simulink model "AdderSubtractor"  (R2014a)
settings: Solver=ode45  StartTime=0.0  StopTime=10.0  RelTol=1e-3  EnableMultiTasking=on
libraries: hdlsllib x17
settings Model: Creator=downing.s  LastModifiedBy=you.r
settings OptimizationCC: SimCompilerOptimization=off
settings DebuggingCC: MergeDetectMultiDrivingBlocksExec=error  FcnCallInpInsideContextMsg=error  FrameProcessingCompatibilityMsg=error  SFExecutionAtInitializationDiag=none
settings HardwareCC: ProdBitPerSizeT=32  ProdBitPerPtrDiffT=32
settings RTWCC: RTWCompilerOptimization=off
settings ConfigComp: CovMetricSettings=dw  CovHtmlReporting=on  CovSaveCumulativeToWorkspaceVar=on  CovSaveSingleToWorkspaceVar=on  CovExternalEMLEnable=off  CovSFcnEnable=off

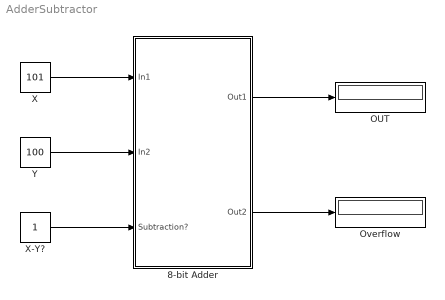
== system AdderSubtractor ==
  8-bit Adder : Subsystem
  OUT : Display
  Overflow : Display
  X : Constant  Value=101  OutDataTypeStr=int8  SampleTime=1
  X-Y? : Constant  OutDataTypeStr=boolean  SampleTime=1
  Y : Constant  Value=100  OutDataTypeStr=int8  SampleTime=1
  wires:
  X/1 -> 8-bit Adder/1(In1)
  Y/1 -> 8-bit Adder/2(In2)
  8-bit Adder/1(Out1) -> OUT/1
  8-bit Adder/2(Out2) -> Overflow/1
  X-Y?/1 -> 8-bit Adder/3("Subtraction? ")

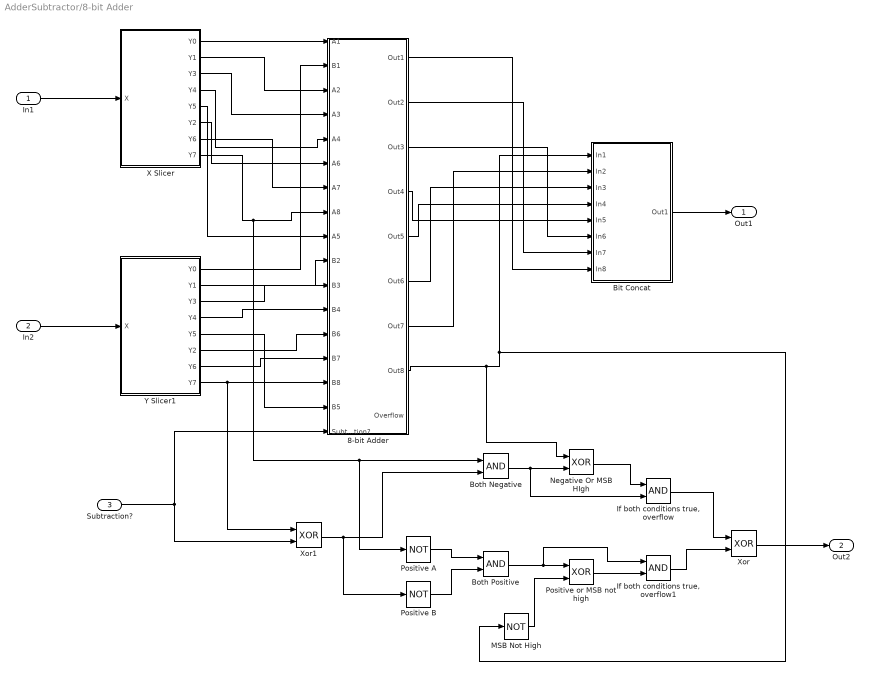
== system AdderSubtractor/8-bit Adder ==
  In1 : Inport
  In2 : Inport  Port=2
  "Subtraction? " : Inport  Port=3
  8-bit Adder : Subsystem
  Bit Concat : Subsystem
  Both Negative : Logic  AllPortsSameDT=off  OutDataTypeStr=boolean
  Both Positive : Logic  AllPortsSameDT=off  OutDataTypeStr=boolean
  "If both conditions true, overflow" : Logic  AllPortsSameDT=off  OutDataTypeStr=boolean
  "If both conditions true, overflow1" : Logic  AllPortsSameDT=off  OutDataTypeStr=boolean
  MSB Not High : Logic  Operator=NOT  AllPortsSameDT=off  OutDataTypeStr=boolean
  Negative Or MSB HIgh : Logic  Operator=XOR  AllPortsSameDT=off  OutDataTypeStr=boolean
  Positive A : Logic  Operator=NOT  AllPortsSameDT=off  OutDataTypeStr=boolean
  Positive B : Logic  Operator=NOT  AllPortsSameDT=off  OutDataTypeStr=boolean
  Positive or MSB not high : Logic  Operator=XOR  AllPortsSameDT=off  OutDataTypeStr=boolean
  X Slicer : Subsystem
  Xor : Logic  Operator=XOR  AllPortsSameDT=off  OutDataTypeStr=boolean
  Xor1 : Logic  Operator=XOR  AllPortsSameDT=off  OutDataTypeStr=boolean
  Y Slicer1 : Subsystem
  Out1 : Outport
  Out2 : Outport  Port=2
  wires:
  Bit Concat/1(Out1) -> Out1/1
  In1/1 -> X Slicer/1(X)
  In2/1 -> Y Slicer1/1(X)
  8-bit Adder/8(Out8) -> Negative Or MSB HIgh/1, MSB Not High/1, Bit Concat/1(In1)
  8-bit Adder/7(Out7) -> Bit Concat/2(In2)
  8-bit Adder/6(Out6) -> Bit Concat/3(In3)
  8-bit Adder/5(Out5) -> Bit Concat/4(In4)
  8-bit Adder/4(Out4) -> Bit Concat/5(In5)
  8-bit Adder/3(Out3) -> Bit Concat/6(In6)
  8-bit Adder/2(Out2) -> Bit Concat/7(In7)
  8-bit Adder/1(Out1) -> Bit Concat/8(In8)
  X Slicer/1(Y0) -> 8-bit Adder/1(A1)
  X Slicer/2(Y1) -> 8-bit Adder/3(A2)
  X Slicer/3(Y3) -> 8-bit Adder/4(A3)
  X Slicer/4(Y4) -> 8-bit Adder/5(A4)
  X Slicer/5(Y5) -> 8-bit Adder/9(A5)
  X Slicer/6(Y2) -> 8-bit Adder/6(A6)
  X Slicer/7(Y6) -> 8-bit Adder/7(A7)
  Y Slicer1/1(Y0) -> 8-bit Adder/2(B1)
  Y Slicer1/2(Y1) -> 8-bit Adder/10(B2)
  Y Slicer1/3(Y3) -> 8-bit Adder/11(B3)
  Y Slicer1/4(Y4) -> 8-bit Adder/12(B4)
  Y Slicer1/5(Y5) -> 8-bit Adder/16(B5)
  Y Slicer1/6(Y2) -> 8-bit Adder/13(B6)
  Y Slicer1/7(Y6) -> 8-bit Adder/14(B7)
  Y Slicer1/8(Y7) -> Xor1/1, 8-bit Adder/15(B8)
  Both Negative/1 -> "If both conditions true, overflow"/2, Negative Or MSB HIgh/2
  Negative Or MSB HIgh/1 -> "If both conditions true, overflow"/1
  X Slicer/8(Y7) -> Positive A/1, Both Negative/1, 8-bit Adder/8(A8)
  Positive A/1 -> Both Positive/1
  Positive B/1 -> Both Positive/2
  Both Positive/1 -> "If both conditions true, overflow1"/1, Positive or MSB not high/1
  MSB Not High/1 -> Positive or MSB not high/2
  Positive or MSB not high/1 -> "If both conditions true, overflow1"/2
  Xor/1 -> Out2/1
  "If both conditions true, overflow1"/1 -> Xor/2
  "If both conditions true, overflow"/1 -> Xor/1
  "Subtraction? "/1 -> 8-bit Adder/17(Subtraction?), Xor1/2
  Xor1/1 -> Positive B/1, Both Negative/2

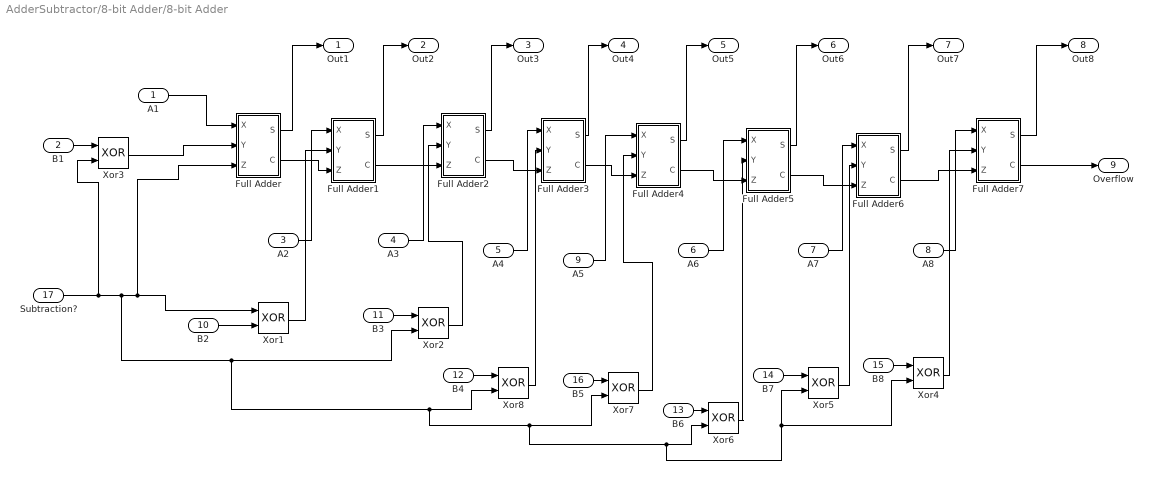
== system AdderSubtractor/8-bit Adder/8-bit Adder ==
  A1 : Inport
  B1 : Inport  Port=2
  A2 : Inport  Port=3
  A3 : Inport  Port=4
  A4 : Inport  Port=5
  A6 : Inport  Port=6
  A7 : Inport  Port=7
  A8 : Inport  Port=8
  A5 : Inport  Port=9
  B2 : Inport  Port=10
  B3 : Inport  Port=11
  B4 : Inport  Port=12
  B6 : Inport  Port=13
  B7 : Inport  Port=14
  B8 : Inport  Port=15
  B5 : Inport  Port=16
  Subtraction? : Inport  Port=17  OutDataTypeStr=boolean
  Full Adder : Subsystem
  Full Adder1 : Subsystem
  Full Adder2 : Subsystem
  Full Adder3 : Subsystem
  Full Adder4 : Subsystem
  Full Adder5 : Subsystem
  Full Adder6 : Subsystem
  Full Adder7 : Subsystem
  Xor{1..8} (8 alike) : Logic  Operator=XOR  AllPortsSameDT=off  OutDataTypeStr=boolean
  Out1 : Outport  OutDataTypeStr=boolean
  Out2 : Outport  Port=2  OutDataTypeStr=boolean
  Out3 : Outport  Port=3  OutDataTypeStr=boolean
  Out4 : Outport  Port=4  OutDataTypeStr=boolean
  Out5 : Outport  Port=5  OutDataTypeStr=boolean
  Out6 : Outport  Port=6  OutDataTypeStr=boolean
  Out7 : Outport  Port=7  OutDataTypeStr=boolean
  Out8 : Outport  Port=8  OutDataTypeStr=boolean
  Overflow : Outport  Port=9  OutDataTypeStr=boolean
  wires:
  Full Adder7/2(C) -> Overflow/1
  Full Adder5/2(C) -> Full Adder6/3(Z)
  Full Adder7/1(S) -> Out8/1
  Full Adder4/2(C) -> Full Adder5/3(Z)
  Full Adder/2(C) -> Full Adder1/3(Z)
  Full Adder6/2(C) -> Full Adder7/3(Z)
  Full Adder6/1(S) -> Out7/1
  Full Adder2/2(C) -> Full Adder3/3(Z)
  Full Adder4/1(S) -> Out5/1
  A2/1 -> Full Adder1/1(X)
  A5/1 -> Full Adder4/1(X)
  Full Adder1/1(S) -> Out2/1
  A7/1 -> Full Adder6/1(X)
  Full Adder5/1(S) -> Out6/1
  A1/1 -> Full Adder/1(X)
  A8/1 -> Full Adder7/1(X)
  A6/1 -> Full Adder5/1(X)
  A4/1 -> Full Adder3/1(X)
  Full Adder3/1(S) -> Out4/1
  Full Adder/1(S) -> Out1/1
  Full Adder1/2(C) -> Full Adder2/3(Z)
  A3/1 -> Full Adder2/1(X)
  Full Adder3/2(C) -> Full Adder4/3(Z)
  Full Adder2/1(S) -> Out3/1
  B2/1 -> Xor1/2
  Subtraction?/1 -> Xor3/2, Xor4/2, Xor5/2, Xor6/2, Xor7/2, Xor8/2, Xor2/2, Full Adder/3(Z), Xor1/1
  Xor1/1 -> Full Adder1/2(Y)
  Xor2/1 -> Full Adder2/2(Y)
  B3/1 -> Xor2/1
  B4/1 -> Xor8/1
  Xor8/1 -> Full Adder3/2(Y)
  B5/1 -> Xor7/1
  Xor7/1 -> Full Adder4/2(Y)
  B6/1 -> Xor6/1
  Xor6/1 -> Full Adder5/2(Y)
  B7/1 -> Xor5/1
  Xor5/1 -> Full Adder6/2(Y)
  Xor4/1 -> Full Adder7/2(Y)
  B8/1 -> Xor4/1
  Xor3/1 -> Full Adder/2(Y)
  B1/1 -> Xor3/1

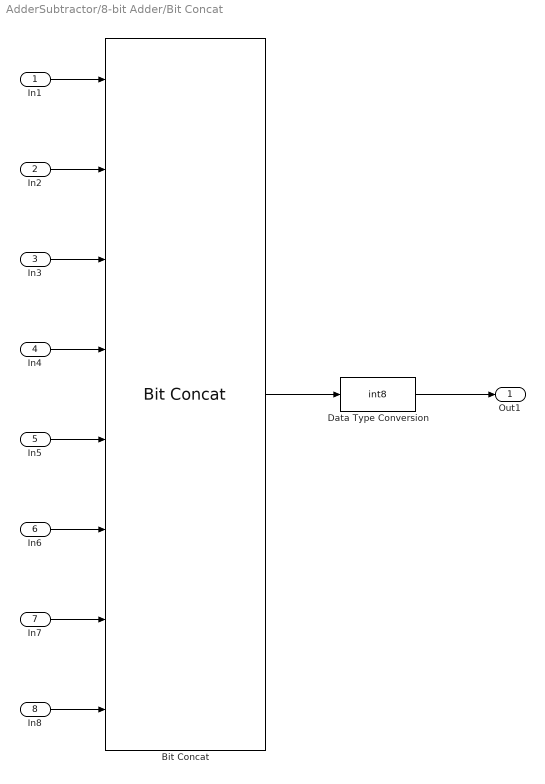
== system AdderSubtractor/8-bit Adder/Bit Concat ==
  In1 : Inport
  In2 : Inport  Port=2
  In3 : Inport  Port=3
  In4 : Inport  Port=4
  In5 : Inport  Port=5
  In6 : Inport  Port=6
  In7 : Inport  Port=7
  In8 : Inport  Port=8
  Bit Concat : hdlsllib/HDL Operations/Bit Concat  numInputs=8
  Data Type Conversion : DataTypeConversion  OutDataTypeStr=int8
  Out1 : Outport
  wires:
  Data Type Conversion/1 -> Out1/1
  In4/1 -> Bit Concat/4
  In1/1 -> Bit Concat/1
  In2/1 -> Bit Concat/2
  In5/1 -> Bit Concat/5
  In6/1 -> Bit Concat/6
  In7/1 -> Bit Concat/7
  In8/1 -> Bit Concat/8
  In3/1 -> Bit Concat/3
  Bit Concat/1 -> Data Type Conversion/1

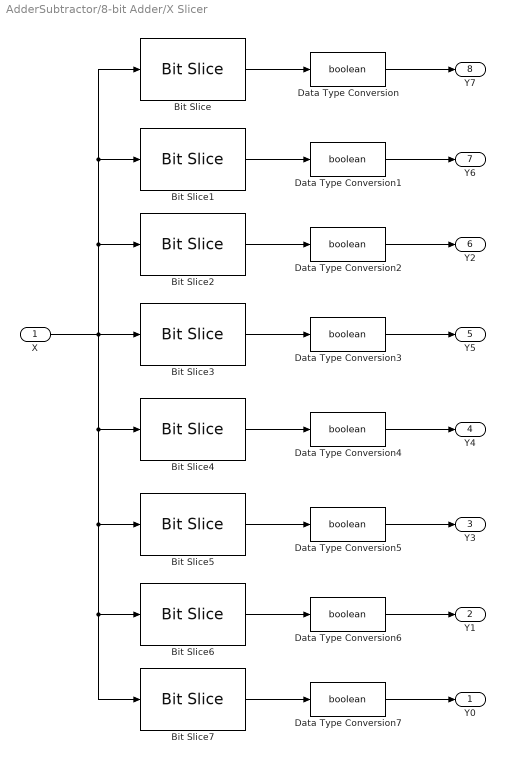
== system AdderSubtractor/8-bit Adder/X Slicer ==
  X : Inport  OutDataTypeStr=int8  SampleTime=1
  Bit Slice : hdlsllib/HDL Operations/Bit Slice  lidx=7  ridx=7
  Bit Slice1 : hdlsllib/HDL Operations/Bit Slice  lidx=6  ridx=6
  Bit Slice2 : hdlsllib/HDL Operations/Bit Slice  lidx=5  ridx=5
  Bit Slice3 : hdlsllib/HDL Operations/Bit Slice  lidx=4  ridx=4
  Bit Slice4 : hdlsllib/HDL Operations/Bit Slice  lidx=3  ridx=3
  Bit Slice5 : hdlsllib/HDL Operations/Bit Slice  lidx=2  ridx=2
  Bit Slice6 : hdlsllib/HDL Operations/Bit Slice  lidx=1  ridx=1
  Bit Slice7 : hdlsllib/HDL Operations/Bit Slice  lidx=0  ridx=0
  Data Type Conversion{,1..7} (8 alike) : DataTypeConversion  OutDataTypeStr=boolean
  Y0 : Outport
  Y1 : Outport  Port=2
  Y3 : Outport  Port=3
  Y4 : Outport  Port=4
  Y5 : Outport  Port=5
  Y2 : Outport  Port=6
  Y6 : Outport  Port=7
  Y7 : Outport  Port=8
  wires:
  X/1 -> Bit Slice4/1, Bit Slice5/1, Bit Slice6/1, Bit Slice7/1, Bit Slice3/1, Bit Slice2/1, Bit Slice1/1, Bit Slice/1
  Data Type Conversion/1 -> Y7/1
  Data Type Conversion1/1 -> Y6/1
  Bit Slice2/1 -> Data Type Conversion2/1
  Bit Slice3/1 -> Data Type Conversion3/1
  Bit Slice4/1 -> Data Type Conversion4/1
  Data Type Conversion6/1 -> Y1/1
  Bit Slice/1 -> Data Type Conversion/1
  Bit Slice1/1 -> Data Type Conversion1/1
  Bit Slice6/1 -> Data Type Conversion6/1
  Data Type Conversion7/1 -> Y0/1
  Bit Slice7/1 -> Data Type Conversion7/1
  Bit Slice5/1 -> Data Type Conversion5/1
  Data Type Conversion2/1 -> Y2/1
  Data Type Conversion3/1 -> Y5/1
  Data Type Conversion4/1 -> Y4/1
  Data Type Conversion5/1 -> Y3/1

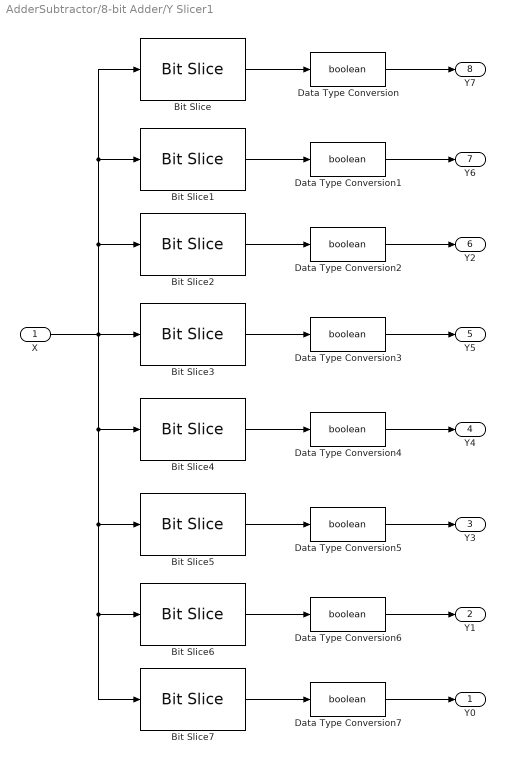
== system AdderSubtractor/8-bit Adder/Y Slicer1 ==
  X : Inport  OutDataTypeStr=int8  SampleTime=1
  Bit Slice : hdlsllib/HDL Operations/Bit Slice  lidx=7  ridx=7
  Bit Slice1 : hdlsllib/HDL Operations/Bit Slice  lidx=6  ridx=6
  Bit Slice2 : hdlsllib/HDL Operations/Bit Slice  lidx=5  ridx=5
  Bit Slice3 : hdlsllib/HDL Operations/Bit Slice  lidx=4  ridx=4
  Bit Slice4 : hdlsllib/HDL Operations/Bit Slice  lidx=3  ridx=3
  Bit Slice5 : hdlsllib/HDL Operations/Bit Slice  lidx=2  ridx=2
  Bit Slice6 : hdlsllib/HDL Operations/Bit Slice  lidx=1  ridx=1
  Bit Slice7 : hdlsllib/HDL Operations/Bit Slice  lidx=0  ridx=0
  Data Type Conversion{,1..7} (8 alike) : DataTypeConversion  OutDataTypeStr=boolean
  Y0 : Outport
  Y1 : Outport  Port=2
  Y3 : Outport  Port=3
  Y4 : Outport  Port=4
  Y5 : Outport  Port=5
  Y2 : Outport  Port=6
  Y6 : Outport  Port=7
  Y7 : Outport  Port=8
  wires:
  X/1 -> Bit Slice4/1, Bit Slice5/1, Bit Slice6/1, Bit Slice7/1, Bit Slice3/1, Bit Slice2/1, Bit Slice1/1, Bit Slice/1
  Data Type Conversion/1 -> Y7/1
  Data Type Conversion1/1 -> Y6/1
  Bit Slice2/1 -> Data Type Conversion2/1
  Bit Slice3/1 -> Data Type Conversion3/1
  Bit Slice4/1 -> Data Type Conversion4/1
  Data Type Conversion6/1 -> Y1/1
  Bit Slice/1 -> Data Type Conversion/1
  Bit Slice1/1 -> Data Type Conversion1/1
  Bit Slice6/1 -> Data Type Conversion6/1
  Data Type Conversion7/1 -> Y0/1
  Bit Slice7/1 -> Data Type Conversion7/1
  Bit Slice5/1 -> Data Type Conversion5/1
  Data Type Conversion2/1 -> Y2/1
  Data Type Conversion3/1 -> Y5/1
  Data Type Conversion4/1 -> Y4/1
  Data Type Conversion5/1 -> Y3/1

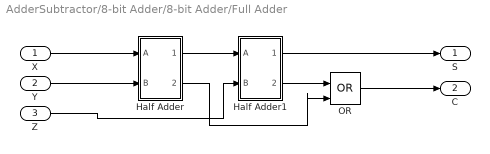
== system AdderSubtractor/8-bit Adder/8-bit Adder/Full Adder ==
  X : Inport
  Y : Inport  Port=2
  Z : Inport  Port=3
  Half Adder : Subsystem
  Half Adder1 : Subsystem
  OR : Logic  Operator=OR  IconShape=distinctive  AllPortsSameDT=off  OutDataTypeStr=boolean
  S : Outport
  C : Outport  Port=2
  wires:
  Half Adder1/1(Sum) -> S/1
  Half Adder/1(Sum) -> Half Adder1/1(A)
  Half Adder/2(Carry) -> OR/2
  X/1 -> Half Adder/1(A)
  Z/1 -> Half Adder1/2(B)
  OR/1 -> C/1
  Y/1 -> Half Adder/2(B)
  Half Adder1/2(Carry) -> OR/1

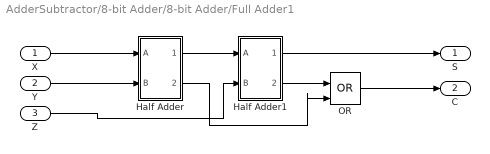
== system AdderSubtractor/8-bit Adder/8-bit Adder/Full Adder1 ==
  X : Inport
  Y : Inport  Port=2
  Z : Inport  Port=3
  Half Adder : Subsystem
  Half Adder1 : Subsystem
  OR : Logic  Operator=OR  IconShape=distinctive  AllPortsSameDT=off  OutDataTypeStr=boolean
  S : Outport
  C : Outport  Port=2
  wires:
  Half Adder1/1(Sum) -> S/1
  Half Adder/1(Sum) -> Half Adder1/1(A)
  Half Adder/2(Carry) -> OR/2
  X/1 -> Half Adder/1(A)
  Z/1 -> Half Adder1/2(B)
  OR/1 -> C/1
  Y/1 -> Half Adder/2(B)
  Half Adder1/2(Carry) -> OR/1

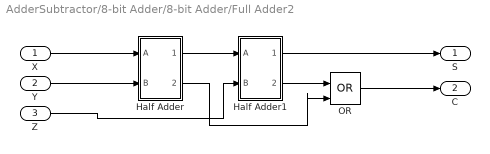
== system AdderSubtractor/8-bit Adder/8-bit Adder/Full Adder2 ==
  X : Inport
  Y : Inport  Port=2
  Z : Inport  Port=3
  Half Adder : Subsystem
  Half Adder1 : Subsystem
  OR : Logic  Operator=OR  IconShape=distinctive  AllPortsSameDT=off  OutDataTypeStr=boolean
  S : Outport
  C : Outport  Port=2
  wires:
  Half Adder1/1(Sum) -> S/1
  Half Adder/1(Sum) -> Half Adder1/1(A)
  Half Adder/2(Carry) -> OR/2
  X/1 -> Half Adder/1(A)
  Z/1 -> Half Adder1/2(B)
  OR/1 -> C/1
  Y/1 -> Half Adder/2(B)
  Half Adder1/2(Carry) -> OR/1

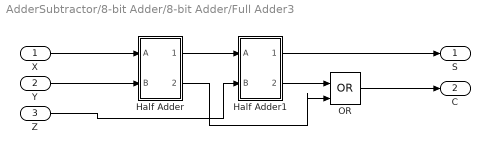
== system AdderSubtractor/8-bit Adder/8-bit Adder/Full Adder3 ==
  X : Inport
  Y : Inport  Port=2
  Z : Inport  Port=3
  Half Adder : Subsystem
  Half Adder1 : Subsystem
  OR : Logic  Operator=OR  IconShape=distinctive  AllPortsSameDT=off  OutDataTypeStr=boolean
  S : Outport
  C : Outport  Port=2
  wires:
  Half Adder1/1(Sum) -> S/1
  Half Adder/1(Sum) -> Half Adder1/1(A)
  Half Adder/2(Carry) -> OR/2
  X/1 -> Half Adder/1(A)
  Z/1 -> Half Adder1/2(B)
  OR/1 -> C/1
  Y/1 -> Half Adder/2(B)
  Half Adder1/2(Carry) -> OR/1

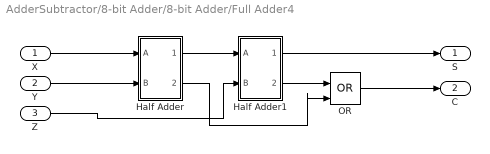
== system AdderSubtractor/8-bit Adder/8-bit Adder/Full Adder4 ==
  X : Inport
  Y : Inport  Port=2
  Z : Inport  Port=3
  Half Adder : Subsystem
  Half Adder1 : Subsystem
  OR : Logic  Operator=OR  IconShape=distinctive  AllPortsSameDT=off  OutDataTypeStr=boolean
  S : Outport
  C : Outport  Port=2
  wires:
  Half Adder1/1(Sum) -> S/1
  Half Adder/1(Sum) -> Half Adder1/1(A)
  Half Adder/2(Carry) -> OR/2
  X/1 -> Half Adder/1(A)
  Z/1 -> Half Adder1/2(B)
  OR/1 -> C/1
  Y/1 -> Half Adder/2(B)
  Half Adder1/2(Carry) -> OR/1

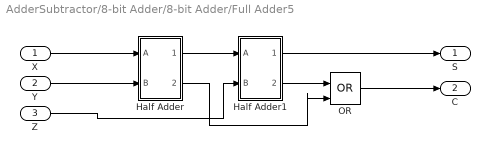
== system AdderSubtractor/8-bit Adder/8-bit Adder/Full Adder5 ==
  X : Inport
  Y : Inport  Port=2
  Z : Inport  Port=3
  Half Adder : Subsystem
  Half Adder1 : Subsystem
  OR : Logic  Operator=OR  IconShape=distinctive  AllPortsSameDT=off  OutDataTypeStr=boolean
  S : Outport
  C : Outport  Port=2
  wires:
  Half Adder1/1(Sum) -> S/1
  Half Adder/1(Sum) -> Half Adder1/1(A)
  Half Adder/2(Carry) -> OR/2
  X/1 -> Half Adder/1(A)
  Z/1 -> Half Adder1/2(B)
  OR/1 -> C/1
  Y/1 -> Half Adder/2(B)
  Half Adder1/2(Carry) -> OR/1

== system AdderSubtractor/8-bit Adder/8-bit Adder/Full Adder6 ==
  X : Inport
  Y : Inport  Port=2
  Z : Inport  Port=3
  Half Adder : Subsystem
  Half Adder1 : Subsystem
  OR : Logic  Operator=OR  IconShape=distinctive  AllPortsSameDT=off  OutDataTypeStr=boolean
  S : Outport
  C : Outport  Port=2
  wires:
  Half Adder1/1(Sum) -> S/1
  Half Adder/1(Sum) -> Half Adder1/1(A)
  Half Adder/2(Carry) -> OR/2
  X/1 -> Half Adder/1(A)
  Z/1 -> Half Adder1/2(B)
  OR/1 -> C/1
  Y/1 -> Half Adder/2(B)
  Half Adder1/2(Carry) -> OR/1

== system AdderSubtractor/8-bit Adder/8-bit Adder/Full Adder7 ==
  X : Inport
  Y : Inport  Port=2
  Z : Inport  Port=3
  Half Adder : Subsystem
  Half Adder1 : Subsystem
  OR : Logic  Operator=OR  IconShape=distinctive  AllPortsSameDT=off  OutDataTypeStr=boolean
  S : Outport
  C : Outport  Port=2
  wires:
  Half Adder1/1(Sum) -> S/1
  Half Adder/1(Sum) -> Half Adder1/1(A)
  Half Adder/2(Carry) -> OR/2
  X/1 -> Half Adder/1(A)
  Z/1 -> Half Adder1/2(B)
  OR/1 -> C/1
  Y/1 -> Half Adder/2(B)
  Half Adder1/2(Carry) -> OR/1

== system AdderSubtractor/8-bit Adder/8-bit Adder/Full Adder/Half Adder ==
  A : Inport
  B : Inport  Port=2
  AND : Logic  IconShape=distinctive  AllPortsSameDT=off  OutDataTypeStr=boolean
  XOR : Logic  Operator=XOR  IconShape=distinctive  AllPortsSameDT=off  OutDataTypeStr=boolean
  Sum : Outport
  Carry : Outport  Port=2
  wires:
  AND/1 -> Carry/1
  XOR/1 -> Sum/1
  B/1 -> XOR/2, AND/2
  A/1 -> AND/1, XOR/1

== system AdderSubtractor/8-bit Adder/8-bit Adder/Full Adder/Half Adder1 ==
  A : Inport
  B : Inport  Port=2
  AND : Logic  IconShape=distinctive  AllPortsSameDT=off  OutDataTypeStr=boolean
  XOR : Logic  Operator=XOR  IconShape=distinctive  AllPortsSameDT=off  OutDataTypeStr=boolean
  Sum : Outport
  Carry : Outport  Port=2
  wires:
  AND/1 -> Carry/1
  XOR/1 -> Sum/1
  B/1 -> XOR/2, AND/2
  A/1 -> AND/1, XOR/1

== system AdderSubtractor/8-bit Adder/8-bit Adder/Full Adder1/Half Adder ==
  A : Inport
  B : Inport  Port=2
  AND : Logic  IconShape=distinctive  AllPortsSameDT=off  OutDataTypeStr=boolean
  XOR : Logic  Operator=XOR  IconShape=distinctive  AllPortsSameDT=off  OutDataTypeStr=boolean
  Sum : Outport
  Carry : Outport  Port=2
  wires:
  AND/1 -> Carry/1
  XOR/1 -> Sum/1
  B/1 -> XOR/2, AND/2
  A/1 -> AND/1, XOR/1

== system AdderSubtractor/8-bit Adder/8-bit Adder/Full Adder1/Half Adder1 ==
  A : Inport
  B : Inport  Port=2
  AND : Logic  IconShape=distinctive  AllPortsSameDT=off  OutDataTypeStr=boolean
  XOR : Logic  Operator=XOR  IconShape=distinctive  AllPortsSameDT=off  OutDataTypeStr=boolean
  Sum : Outport
  Carry : Outport  Port=2
  wires:
  AND/1 -> Carry/1
  XOR/1 -> Sum/1
  B/1 -> XOR/2, AND/2
  A/1 -> AND/1, XOR/1

== system AdderSubtractor/8-bit Adder/8-bit Adder/Full Adder2/Half Adder ==
  A : Inport
  B : Inport  Port=2
  AND : Logic  IconShape=distinctive  AllPortsSameDT=off  OutDataTypeStr=boolean
  XOR : Logic  Operator=XOR  IconShape=distinctive  AllPortsSameDT=off  OutDataTypeStr=boolean
  Sum : Outport
  Carry : Outport  Port=2
  wires:
  AND/1 -> Carry/1
  XOR/1 -> Sum/1
  B/1 -> XOR/2, AND/2
  A/1 -> AND/1, XOR/1

== system AdderSubtractor/8-bit Adder/8-bit Adder/Full Adder2/Half Adder1 ==
  A : Inport
  B : Inport  Port=2
  AND : Logic  IconShape=distinctive  AllPortsSameDT=off  OutDataTypeStr=boolean
  XOR : Logic  Operator=XOR  IconShape=distinctive  AllPortsSameDT=off  OutDataTypeStr=boolean
  Sum : Outport
  Carry : Outport  Port=2
  wires:
  AND/1 -> Carry/1
  XOR/1 -> Sum/1
  B/1 -> XOR/2, AND/2
  A/1 -> AND/1, XOR/1

== system AdderSubtractor/8-bit Adder/8-bit Adder/Full Adder3/Half Adder ==
  A : Inport
  B : Inport  Port=2
  AND : Logic  IconShape=distinctive  AllPortsSameDT=off  OutDataTypeStr=boolean
  XOR : Logic  Operator=XOR  IconShape=distinctive  AllPortsSameDT=off  OutDataTypeStr=boolean
  Sum : Outport
  Carry : Outport  Port=2
  wires:
  AND/1 -> Carry/1
  XOR/1 -> Sum/1
  B/1 -> XOR/2, AND/2
  A/1 -> AND/1, XOR/1

== system AdderSubtractor/8-bit Adder/8-bit Adder/Full Adder3/Half Adder1 ==
  A : Inport
  B : Inport  Port=2
  AND : Logic  IconShape=distinctive  AllPortsSameDT=off  OutDataTypeStr=boolean
  XOR : Logic  Operator=XOR  IconShape=distinctive  AllPortsSameDT=off  OutDataTypeStr=boolean
  Sum : Outport
  Carry : Outport  Port=2
  wires:
  AND/1 -> Carry/1
  XOR/1 -> Sum/1
  B/1 -> XOR/2, AND/2
  A/1 -> AND/1, XOR/1

== system AdderSubtractor/8-bit Adder/8-bit Adder/Full Adder4/Half Adder ==
  A : Inport
  B : Inport  Port=2
  AND : Logic  IconShape=distinctive  AllPortsSameDT=off  OutDataTypeStr=boolean
  XOR : Logic  Operator=XOR  IconShape=distinctive  AllPortsSameDT=off  OutDataTypeStr=boolean
  Sum : Outport
  Carry : Outport  Port=2
  wires:
  AND/1 -> Carry/1
  XOR/1 -> Sum/1
  B/1 -> XOR/2, AND/2
  A/1 -> AND/1, XOR/1

== system AdderSubtractor/8-bit Adder/8-bit Adder/Full Adder4/Half Adder1 ==
  A : Inport
  B : Inport  Port=2
  AND : Logic  IconShape=distinctive  AllPortsSameDT=off  OutDataTypeStr=boolean
  XOR : Logic  Operator=XOR  IconShape=distinctive  AllPortsSameDT=off  OutDataTypeStr=boolean
  Sum : Outport
  Carry : Outport  Port=2
  wires:
  AND/1 -> Carry/1
  XOR/1 -> Sum/1
  B/1 -> XOR/2, AND/2
  A/1 -> AND/1, XOR/1

== system AdderSubtractor/8-bit Adder/8-bit Adder/Full Adder5/Half Adder ==
  A : Inport
  B : Inport  Port=2
  AND : Logic  IconShape=distinctive  AllPortsSameDT=off  OutDataTypeStr=boolean
  XOR : Logic  Operator=XOR  IconShape=distinctive  AllPortsSameDT=off  OutDataTypeStr=boolean
  Sum : Outport
  Carry : Outport  Port=2
  wires:
  AND/1 -> Carry/1
  XOR/1 -> Sum/1
  B/1 -> XOR/2, AND/2
  A/1 -> AND/1, XOR/1

== system AdderSubtractor/8-bit Adder/8-bit Adder/Full Adder5/Half Adder1 ==
  A : Inport
  B : Inport  Port=2
  AND : Logic  IconShape=distinctive  AllPortsSameDT=off  OutDataTypeStr=boolean
  XOR : Logic  Operator=XOR  IconShape=distinctive  AllPortsSameDT=off  OutDataTypeStr=boolean
  Sum : Outport
  Carry : Outport  Port=2
  wires:
  AND/1 -> Carry/1
  XOR/1 -> Sum/1
  B/1 -> XOR/2, AND/2
  A/1 -> AND/1, XOR/1

== system AdderSubtractor/8-bit Adder/8-bit Adder/Full Adder6/Half Adder ==
  A : Inport
  B : Inport  Port=2
  AND : Logic  IconShape=distinctive  AllPortsSameDT=off  OutDataTypeStr=boolean
  XOR : Logic  Operator=XOR  IconShape=distinctive  AllPortsSameDT=off  OutDataTypeStr=boolean
  Sum : Outport
  Carry : Outport  Port=2
  wires:
  AND/1 -> Carry/1
  XOR/1 -> Sum/1
  B/1 -> XOR/2, AND/2
  A/1 -> AND/1, XOR/1

== system AdderSubtractor/8-bit Adder/8-bit Adder/Full Adder6/Half Adder1 ==
  A : Inport
  B : Inport  Port=2
  AND : Logic  IconShape=distinctive  AllPortsSameDT=off  OutDataTypeStr=boolean
  XOR : Logic  Operator=XOR  IconShape=distinctive  AllPortsSameDT=off  OutDataTypeStr=boolean
  Sum : Outport
  Carry : Outport  Port=2
  wires:
  AND/1 -> Carry/1
  XOR/1 -> Sum/1
  B/1 -> XOR/2, AND/2
  A/1 -> AND/1, XOR/1

== system AdderSubtractor/8-bit Adder/8-bit Adder/Full Adder7/Half Adder ==
  A : Inport
  B : Inport  Port=2
  AND : Logic  IconShape=distinctive  AllPortsSameDT=off  OutDataTypeStr=boolean
  XOR : Logic  Operator=XOR  IconShape=distinctive  AllPortsSameDT=off  OutDataTypeStr=boolean
  Sum : Outport
  Carry : Outport  Port=2
  wires:
  AND/1 -> Carry/1
  XOR/1 -> Sum/1
  B/1 -> XOR/2, AND/2
  A/1 -> AND/1, XOR/1

== system AdderSubtractor/8-bit Adder/8-bit Adder/Full Adder7/Half Adder1 ==
  A : Inport
  B : Inport  Port=2
  AND : Logic  IconShape=distinctive  AllPortsSameDT=off  OutDataTypeStr=boolean
  XOR : Logic  Operator=XOR  IconShape=distinctive  AllPortsSameDT=off  OutDataTypeStr=boolean
  Sum : Outport
  Carry : Outport  Port=2
  wires:
  AND/1 -> Carry/1
  XOR/1 -> Sum/1
  B/1 -> XOR/2, AND/2
  A/1 -> AND/1, XOR/1
